simulink model "slx_Pendulum_Discreto_Cascade"  (R2023a)
settings: Solver=ode45  StartTime=0  StopTime=simulation_T_f  MaxStep=MaxStep  RelTol=RelTol  AbsTol=1e-6
values from neighbouring files (symbols this model uses):
  A_alpha_angle = I_angle + Ts * (I_angle - alpha_angle * A_CTRL_angle * Ts)^-1 * A_CTRL_angle    [Tesi_DiscretoCascade.m]    (also in tesi_sperimentale.m)
  B_alpha_1_angle = (1 - alpha_angle) * Ts * (I_angle - alpha_angle * A_CTRL_angle * Ts)^-1 * B_CTRL_angle    [Tesi_DiscretoCascade.m]    (also in tesi_sperimentale.m)
  B_alpha_2_angle = alpha_angle * Ts * (I_angle - alpha_angle * A_CTRL_angle * Ts)^-1 * B_CTRL_angle    [Tesi_DiscretoCascade.m]    (also in tesi_sperimentale.m)
  C_CTRL_angle = f_KR_angle_LTI.C    [Tesi_DiscretoCascade.m]    (also in tesi_sperimentale.m)
  C_CTRL_position = f_KR_position_LTI.C    [Tesi_DiscretoCascade.m]    (also in tesi_sperimentale.m)
  cascade_A_alpha_position = cascade_I_position + Ts * (cascade_I_position - cascade_alpha_position * A_CTRL_position * Ts)^-1 * A_CTRL_position    [Tesi_DiscretoCascade.m]    (also in tesi_sperimentale.m)
  cascade_B_alpha_1_position = (1 - cascade_alpha_position) * Ts * (cascade_I_position - cascade_alpha_position * A_CTRL_position * Ts)^-1 * B_CTRL_position    [Tesi_DiscretoCascade.m]    (also in tesi_sperimentale.m)
  cascade_B_alpha_2_position = cascade_alpha_position * Ts * (cascade_I_position - cascade_alpha_position * A_CTRL_position * Ts)^-1 * B_CTRL_position    [Tesi_DiscretoCascade.m]    (also in tesi_sperimentale.m)
  D_CTRL_angle = f_KR_angle_LTI.D    [Tesi_DiscretoCascade.m]    (also in tesi_sperimentale.m)
  D_CTRL_position = f_KR_position_LTI.D    [Tesi_DiscretoCascade.m]    (also in tesi_sperimentale.m)
  init_omega0 = 0    [Tesi_DiscretoCascade.m]    (also in tesi_sperimentale.m)
  init_positionRef = 0    [Tesi_DiscretoCascade.m]    (also in tesi_sperimentale.m)
  init_theta0 = pi/12    (= 0.261799387799)    [Tesi_DiscretoCascade.m]    (also in tesi_sperimentale.m)
  init_thetaRef = 0    [Tesi_DiscretoCascade.m]    (also in tesi_sperimentale.m)
  init_v0 = 0    [Tesi_DiscretoCascade.m]    (also in tesi_sperimentale.m)
  init_x0 = -3    [Tesi_DiscretoCascade.m]    (also in tesi_sperimentale.m)
  p_b = 0.1    [Tesi_DiscretoCascade.m]    (also in tesi_sperimentale.m)
  p_g = 9.81    [Tesi_DiscretoCascade.m]    (also in tesi_sperimentale.m)
  p_Ja = (1/12)*p_ma*p_l^2    (= 0.0019575)    [Tesi_DiscretoCascade.m]    (also in tesi_sperimentale.m)
  p_Jb = 0    [Tesi_DiscretoCascade.m]    (also in tesi_sperimentale.m)
  p_k = 0    [Tesi_DiscretoCascade.m]    (also in tesi_sperimentale.m)
  p_l = 0.45    [Tesi_DiscretoCascade.m]    (also in tesi_sperimentale.m)
  p_M = 0.61    [Tesi_DiscretoCascade.m]    (also in tesi_sperimentale.m)
  p_ma = 0.116    [Tesi_DiscretoCascade.m]    (also in tesi_sperimentale.m)
  p_mb = 0.05    [Tesi_DiscretoCascade.m]    (also in tesi_sperimentale.m)
  Ts = 0.002    [Tesi_DiscretoCascade.m]    (also in tesi_sperimentale.m)
Description:
  | Inverted Pendulum with Animation
  | 
  | This example shows how to model an inverted pendulum.  The animation is created using MATLAB(R) Handle Graphics(R).  The animation block is a masked
  | S-function.  For more information, use the context menu to look under the Animation block's mask
  | and open the S-function for editing.
settings Model: Creator=The MathWorks, Inc.  LastModifiedBy=admin
settings SolverCC: AutoScaleAbsTol=off  AlgebraicLoopSolver=TrustRegion
settings DataIOCC: ExternalInput=[]  InitialState=[]  SaveFormat=Array  SaveOutput=off  SaveTime=off  ReturnWorkspaceOutputs=off
settings OptimizationCC: BlockReduction=off  BooleanDataType=off  ReuseModelBlockBuffer=off  ExpressionDepthLimit=2147483647  InitFltsAndDblsToZero=on  LifeSpan=inf
settings DebuggingCC: SaveWithParameterizedLinksMsg=none  UnderspecifiedInitializationDetection=Classic  MergeDetectMultiDrivingBlocksExec=none  SignalResolutionControl=TryResolveAllWithWarning  MultiTaskDSMMsg=warning  MultiTaskCondExecSysMsg=none  SigSpecEnsureSampleTimeMsg=none  FcnCallInpInsideContextMsg=warning  UnconnectedInputMsg=warning  UnconnectedOutputMsg=warning  UnconnectedLineMsg=warning  StateNameClashWarn=warning  SFUnexpectedBacktrackingDiag=warning  SFNoUnconditionalDefaultTransitionDiag=warning  SFExecutionAtInitializationDiag=none  ArithmeticOperatorsInVariantConditions=warning
settings HardwareCC: ProdBitPerPointer=32  ProdBitPerSizeT=32  ProdBitPerPtrDiffT=32  ProdLargestAtomicFloat=None  ProdIntDivRoundTo=Undefined  ProdEndianess=Unspecified  ProdWordSize=32  ProdHWDeviceType=32-bit Generic  TargetUnknown=on
settings ModelReferenceCC: EnableRefExpFcnMdlSchedulingChecks=on  PropagateSignalLabelsOutOfModel=off
settings SFSimCC: SimUseLocalCustomCode=off  CustomCodeUndefinedFunction=UseInterfaceOnly
settings RTWCC: RTWUseLocalCustomCode=off
settings CodeAppCC: StateflowObjectComments=on
settings GRTTargetCC: TargetFcnLib=ansi_tfl_tmw.mat  TargetLangStandard=C89/C90 (ANSI)  CombineOutputUpdateFcns=off  GRTInterface=on
settings ConfigComp: CovMetricSettings=dw  CovSaveCumulativeToWorkspaceVar=on  CovSaveSingleToWorkspaceVar=on  CovExternalEMLEnable=off

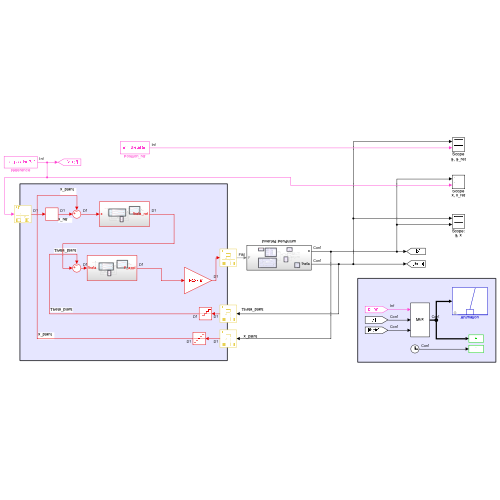
[thumbnail: Simulink's stored preview of the top-level diagram]
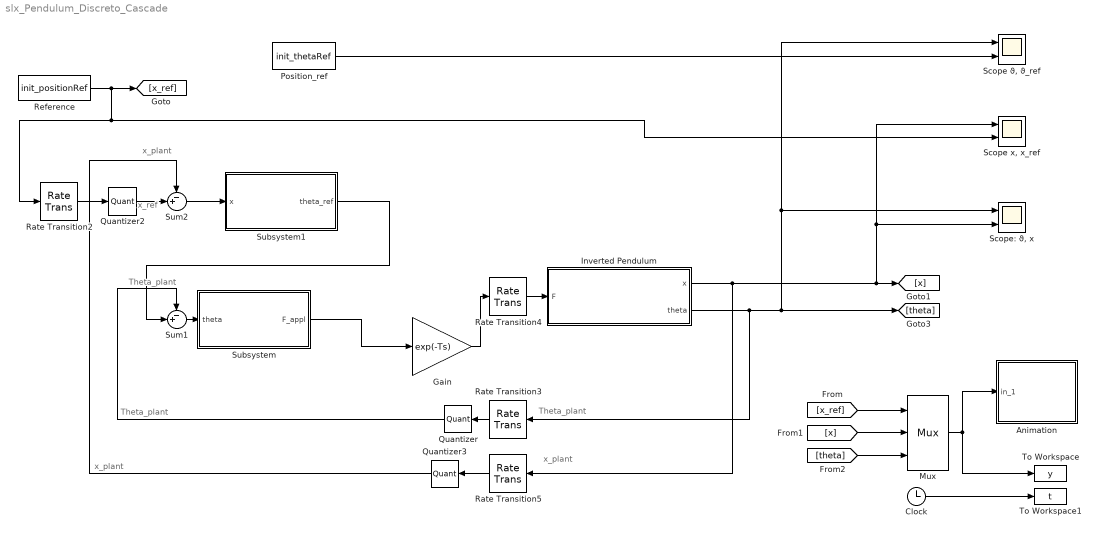
== system slx_Pendulum_Discreto_Cascade ==
  note: Theta_plant
  note: x_plant
  note: x_ref
  note: Theta_plant
  note: x_plant
  note: Theta_plant
  note: x_plant
  Animation : Subsystem  mask(Pendulum plot){RefBlock=Reference}
      mask prompts: RefBlock "DC reference signal block name:"
      mask help: Pendulum plot
      mask Help: Pendulum animation function using Handle graphics.
      mask Display: plot([-10 10],[0 0],[-2 -2 2 2],[0 1 1 0],[0 3],[1 5])
  Clock : Clock
  Gain : Gain  Gain=exp(-Ts)
  Inverted Pendulum : Subsystem
  Mux : Mux  Inputs=3
  Position_ref : Constant  Value=init_thetaRef
  Quantizer : Quantizer  QuantizationInterval=2*pi/2^15
  Quantizer2 : Quantizer  QuantizationInterval=2*pi/2^15
  Quantizer3 : Quantizer  QuantizationInterval=2*pi/2^15
  Rate Transition2 : RateTransition  Integrity=off  OutPortSampleTime=Ts
  Rate Transition3 : RateTransition  Integrity=off  OutPortSampleTime=Ts
  Rate Transition4 : RateTransition  Integrity=off  OutPortSampleTime=0
  Rate Transition5 : RateTransition  Integrity=off  OutPortSampleTime=Ts
  Reference : Constant  Value=init_positionRef
  "Scope x, x_ref" : Scope  NumInputPorts=2
  "Scope ϑ, ϑ_ref" : Scope  NumInputPorts=2
  "Scope: ϑ, x" : Scope  NumInputPorts=2
  Subsystem : Subsystem
  Subsystem1 : Subsystem
  Sum1 : Sum  Inputs=-+|
  Sum2 : Sum  Inputs=-+|
  To Workspace : ToWorkspace  VariableName=y  SampleTime=0.02
  To Workspace1 : ToWorkspace  VariableName=t  SampleTime=0.02
  wires:
  [x_ref] -> Mux/1
  [x] -> Mux/2
  [theta] -> Mux/3
  Mux/1 -> To Workspace/1, Animation/1(in_1)
  Clock/1 -> To Workspace1/1
  Inverted Pendulum/1(x) -> Rate Transition5/1, "Scope x, x_ref"/1, "Scope: ϑ, x"/2, [x]
  Inverted Pendulum/2(theta) -> "Scope ϑ, ϑ_ref"/1, "Scope: ϑ, x"/1, [theta], Rate Transition3/1
  Rate Transition4/1 -> Inverted Pendulum/1(F)
  Rate Transition3/1 -> Quantizer/1
  Quantizer/1 -> Sum1/1
  Sum1/1 -> Subsystem/1(theta)
  Reference/1 -> [x_ref], "Scope x, x_ref"/2, Rate Transition2/1
  Rate Transition2/1 -> Quantizer2/1
  Quantizer2/1 -> Sum2/2
  Rate Transition5/1 -> Quantizer3/1
  Quantizer3/1 -> Sum2/1
  Subsystem1/1(theta_ref) -> Sum1/2
  Sum2/1 -> Subsystem1/1(x)
  Gain/1 -> Rate Transition4/1
  Position_ref/1 -> "Scope ϑ, ϑ_ref"/2
  Subsystem/1(F_appl) -> Gain/1

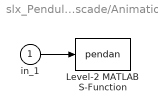
== system slx_Pendulum_Discreto_Cascade/Animation ==
  in_1 : Inport
  Level-2 MATLAB S-Function : M-S-Function  FunctionName=pendan  Parameters=RefBlock
  wires:
  in_1/1 -> Level-2 MATLAB S-Function/1

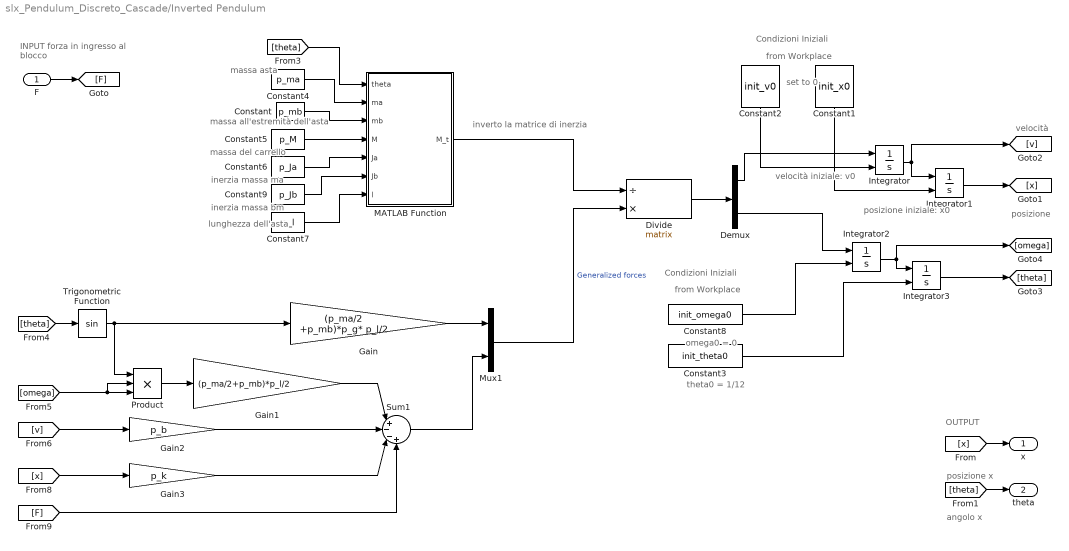
== system slx_Pendulum_Discreto_Cascade/Inverted Pendulum ==
  note: from Workplace
  note: posizione x
  note: inverto la matrice di inerzia
  note: inerzia massa ma
  note: massa del carrello
  note: massa asta
  note: INPUT
      | forza in ingresso al blocco
  note: massa all'estremità
      | dell'asta
  note: inerzia massa bm
  note: lunghezza dell'asta
  note: OUTPUT
  note: angolo x
  note: theta0 = 1/12
  note: omega0 = 0
  note: from Workplace
  note: set to 0
  note: Condizioni Iniziali
  note: velocità
  note: posizione
  note: Condizioni Iniziali
  note: velocità iniziale: v0
  note: posizione iniziale: x0
  F : Inport
  Constant : Constant  Value=p_mb
  Constant1 : Constant  Value=init_x0
  Constant2 : Constant  Value=init_v0
  Constant3 : Constant  Value=init_theta0
  Constant4 : Constant  Value=p_ma
  Constant5 : Constant  Value=p_M
  Constant6 : Constant  Value=p_Ja
  Constant7 : Constant  Value=p_l
  Constant8 : Constant  Value=init_omega0
  Constant9 : Constant  Value=p_Jb
  Demux : Demux  Outputs=2
  Divide : Product  Inputs=/*  Multiplication=Matrix(*)
  Gain : Gain  Gain=(p_ma/2 +p_mb)*p_g* p_l/2
  Gain1 : Gain  Gain=(p_ma/2+p_mb)*p_l/2
  Gain2 : Gain  Gain=p_b
  Gain3 : Gain  Gain=p_k
  Integrator : Integrator  InitialConditionSource=external
  Integrator1 : Integrator  InitialConditionSource=external
  Integrator2 : Integrator  InitialConditionSource=external
  Integrator3 : Integrator  InitialConditionSource=external  WrapState=on
  MATLAB Function : MATLAB Function  TreatAsAtomicUnit=on
  Mux1 : Mux  Inputs=2
  Product : Product  Inputs=3
  Sum1 : Sum  Inputs=|+--+
  Trigonometric Function : Trigonometry
  x : Outport
  theta : Outport  Port=2
  wires:
  Integrator/1 -> [v], Integrator1/1
  Integrator3/1 -> [theta]
  [omega] -> Product/2, Product/3
  Integrator1/1 -> [x]
  Integrator2/1 -> Integrator3/1, [omega]
  Divide/1 -> Demux/1
  Demux/2 -> Integrator2/1
  Gain2/1 -> Sum1/2
  Sum1/1 -> Mux1/2
  [theta] -> Trigonometric Function/1
  Product/1 -> Gain1/1
  MATLAB Function/1(M_t) -> Divide/1
  Gain/1 -> Mux1/1
  Trigonometric Function/1 -> Gain/1, Product/1
  Mux1/1 -> Divide/2  "Generalized forces"
  [F] -> Sum1/4
  Gain1/1 -> Sum1/1
  Constant2/1 -> Integrator/2
  Constant3/1 -> Integrator3/2
  [x] -> Gain3/1
  Demux/1 -> Integrator/1
  Gain3/1 -> Sum1/3
  [v] -> Gain2/1
  Constant1/1 -> Integrator1/2
  F/1 -> [F]
  [x] -> x/1
  [theta] -> theta/1
  Constant8/1 -> Integrator2/2
  [theta] -> MATLAB Function/1(theta)
  Constant4/1 -> MATLAB Function/2(ma)
  Constant5/1 -> MATLAB Function/4(M)
  Constant/1 -> MATLAB Function/3(mb)
  Constant6/1 -> MATLAB Function/5(Ja)
  Constant9/1 -> MATLAB Function/6(Jb)
  Constant7/1 -> MATLAB Function/7(l)

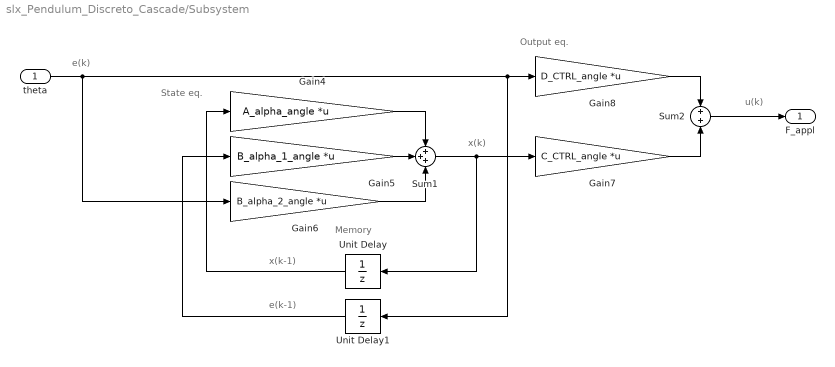
== system slx_Pendulum_Discreto_Cascade/Subsystem ==
  note: x(k)
  note: u(k)
  note: x(k-1)
  note: e(k-1)
  note: e(k)
  note: Memory
  note: State eq.
  note: Output eq.
  theta : Inport
  Gain4 : Gain  Gain=A_alpha_angle  Multiplication=Matrix(K*u)
  Gain5 : Gain  Gain=B_alpha_1_angle  Multiplication=Matrix(K*u)
  Gain6 : Gain  Gain=B_alpha_2_angle  Multiplication=Matrix(K*u)
  Gain7 : Gain  Gain=C_CTRL_angle  Multiplication=Matrix(K*u)
  Gain8 : Gain  Gain=D_CTRL_angle  Multiplication=Matrix(K*u)
  Sum1 : Sum  Inputs=+++
  Sum2 : Sum
  Unit Delay : UnitDelay  SampleTime=Ts  HasFrameUpgradeWarning=on
  Unit Delay1 : UnitDelay  SampleTime=Ts  HasFrameUpgradeWarning=on
  F_appl : Outport
  wires:
  theta/1 -> Gain8/1, Unit Delay1/1, Gain6/1
  Unit Delay/1 -> Gain4/1
  Sum1/1 -> Unit Delay/1, Gain7/1
  Sum2/1 -> F_appl/1
  Gain6/1 -> Sum1/3
  Gain7/1 -> Sum2/2
  Gain5/1 -> Sum1/2
  Gain4/1 -> Sum1/1
  Gain8/1 -> Sum2/1
  Unit Delay1/1 -> Gain5/1

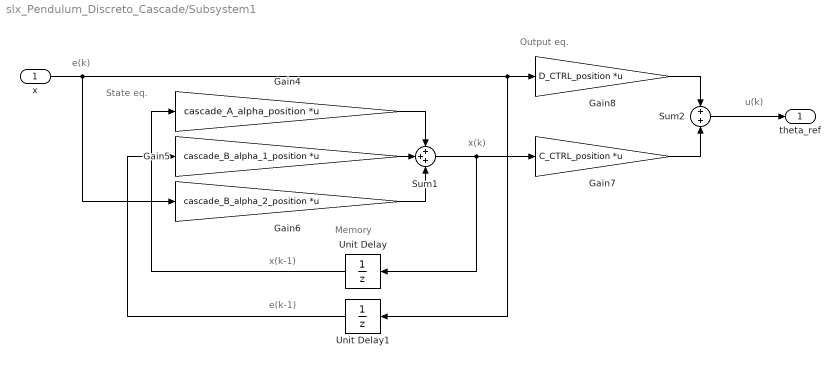
== system slx_Pendulum_Discreto_Cascade/Subsystem1 ==
  note: State eq.
  note: x(k)
  note: Memory
  note: u(k)
  note: Output eq.
  note: e(k-1)
  note: x(k-1)
  note: e(k)
  x : Inport
  Gain4 : Gain  Gain=cascade_A_alpha_position  Multiplication=Matrix(K*u)
  Gain5 : Gain  Gain=cascade_B_alpha_1_position  Multiplication=Matrix(K*u)
  Gain6 : Gain  Gain=cascade_B_alpha_2_position  Multiplication=Matrix(K*u)
  Gain7 : Gain  Gain=C_CTRL_position  Multiplication=Matrix(K*u)
  Gain8 : Gain  Gain=D_CTRL_position  Multiplication=Matrix(K*u)
  Sum1 : Sum  Inputs=+++
  Sum2 : Sum
  Unit Delay : UnitDelay  SampleTime=Ts  HasFrameUpgradeWarning=on
  Unit Delay1 : UnitDelay  SampleTime=Ts  HasFrameUpgradeWarning=on
  theta_ref : Outport
  wires:
  Gain4/1 -> Sum1/1
  Sum1/1 -> Unit Delay/1, Gain7/1
  Unit Delay/1 -> Gain4/1
  Gain7/1 -> Sum2/2
  x/1 -> Gain8/1, Unit Delay1/1, Gain6/1
  Gain6/1 -> Sum1/3
  Gain5/1 -> Sum1/2
  Gain8/1 -> Sum2/1
  Unit Delay1/1 -> Gain5/1
  Sum2/1 -> theta_ref/1

== matlab function slx_Pendulum_Discreto_Cascade/Inverted Pendulum/MATLAB Function ==
  data: theta input; M_t output; ma input; mb input; M input; Ja input; Jb input; l input
function M_t = Inertia(theta, ma, mb, M, Ja, Jb, l)
%% Computation of the inertia matrix
M_t = [(ma/2+mb)*l*cos(theta) (ma/4+mb)*l^2+Ja+Jb;
            M+ma+mb (ma/2+mb)*l*cos(theta)];
